simulink model "fig2_4_simulink"  (R2021b)
settings: Solver=ode45  StartTime=0.0  StopTime=3  RelTol=1e-3  EnableMultiTasking=on
model workspace (MAT data in the model file):
  X0 = 0
settings Model: Creator=One Informatic  LastModifiedBy=One Informatic
settings DataIOCC: LimitDataPoints=on  SaveFormat=Array  SignalLoggingSaveFormat=ModelDataLogs  ReturnWorkspaceOutputs=off  SignalLoggingName=sigsOut
settings DebuggingCC: SaveWithParameterizedLinksMsg=none  UnderspecifiedInitializationDetection=Classic  MergeDetectMultiDrivingBlocksExec=none  SignalResolutionControl=TryResolveAllWithWarning  MultiTaskDSMMsg=warning  MultiTaskCondExecSysMsg=none
settings HardwareCC: ProdBitPerPointer=32  ProdBitPerSizeT=32  ProdBitPerPtrDiffT=32  ProdLargestAtomicFloat=None  ProdIntDivRoundTo=Undefined  ProdEndianess=Unspecified  ProdWordSize=32  ProdHWDeviceType=32-bit Generic  TargetUnknown=on
settings ModelReferenceCC: PropagateSignalLabelsOutOfModel=off
settings GRTTargetCC: CombineOutputUpdateFcns=off  GRTInterface=on
settings ConfigComp: CovMetricSettings=dw  CovSaveCumulativeToWorkspaceVar=on  CovSaveSingleToWorkspaceVar=on

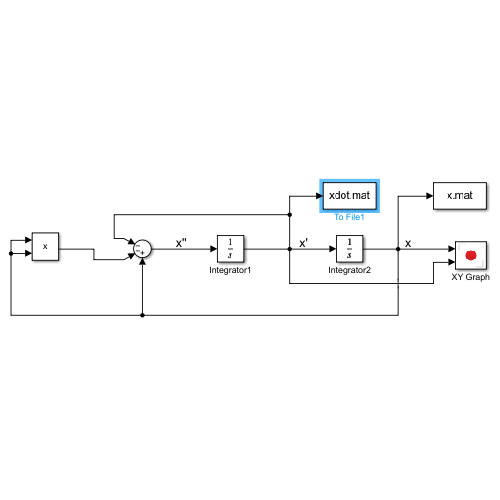
[thumbnail: Simulink's stored preview of the top-level diagram]
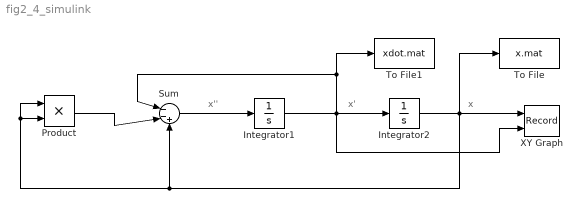
== system fig2_4_simulink ==
  note: x''
  note: x'
  note: x
  Integrator1 : Integrator  InitialCondition=1.5
  Integrator2 : Integrator  InitialCondition=-1
  Product : Product
  Sum : Sum  Inputs=|--+
  To File : ToFile  Filename=x.mat  MatrixName=x  SampleTime=0.001
  To File1 : ToFile  Filename=xdot.mat  MatrixName=xdot  SampleTime=0.001
  XY Graph : Record  FileSettingsInternal="{\"entries\":[{\"content\":{\"excelSettings\":{\"content\":{},\"type\":\"Streamout.ExcelSettings\"}},\"type\":\"Streamout.FileSettingStorage\",\"uuid\":\"c2565e3c-df81-4bf1-9553-0a324edf4095\"}],\"packageUris\":[\"http://schema.mathworks.com/mf0/streamout_blocks/R2020a\"],\"version\":\"1.0\"}"  Layout=[1 1]  SignalsInternal="{\"entries\":[{\"content\":{\"signals\":[{\"content\":{\"blockPath\":[\"fig2_4_simulink/XY Graph\"],\"channel\":[],\"dimensions\":[1],\"domain\":\"fig2_4_simulink/XY Graph\",\"lineColor\":\"#a2142f\",\"plots\":[1],\"port\":1,\"sid\":[\"\"],\"signalID\":974,\"signalName\":\"Integrator2\"},\"type\":\"RecordBlkView.Signal\",\"uuid\":\"0da2719f-7509-43da-93cb-1d4f29ef6b94\"},{\"content\":{\"blockPath\":[\"fig2_4_simulink/XY Graph\"],\"channel\":[],\"dimensions\":[1],\"domain\":\"fig2_4_simulink/XY Graph\",\"lineColor\":\"#139fff\",\"plots\":[1],\"port\":2,\"sid\":[\"\"],\"signalID\":978,\"signalName\":\"Integrator1\"},\"type\":\"RecordBlkView.Signal\",\"uuid\":\"15e696ae-383a-4cf5-bb14-1c1c06f9cb84\"}]},\"type\":\"RecordBlkView.InputSignals\",\"uuid\":\"ba74110e-d626-4785-bf17-a2d6001b194a\"}],\"packageUris\":[\"http://schema.mathworks.com/mf0/streamout_blocks/R2020a\"],\"version\":\"1.0\"}"  VisualizationBindings="{\"xyplotplugin\":{\"info\":[{\"series\":[{\"bindingParametersList\":[{\"parameter\":\"X-Axis\",\"signalID\":974,\"signalName\":\"Integrator2\"},{\"parameter\":\"Y-Axis\",\"signalID\":978,\"signalName\":\"Integrator1\"}],\"seriesID\":8348}],\"subplotID\":1}]}}"  CompatibilityTag=XY
  wires:
  Product/1 -> Sum/2
  Sum/1 -> Integrator1/1
  Integrator2/1 -> Product/1, Product/2, Sum/3, To File/1, XY Graph/1
  Integrator1/1 -> To File1/1, Sum/1, XY Graph/2, Integrator2/1
